simulink model "drone_sim"  (R2022b)
settings: Solver=VariableStepAuto  StartTime=0.0  StopTime=10  RelTol=1e-3
values from neighbouring files (symbols this model uses):
  attitude_0 = [pi/2;pi/2;pi/2;1]    [drone.m]
  g = 9.81    [drone.m]
  k = 1    [drone.m]
  p0 = [0;0;0]    [drone.m]    (also in drone_2.m)
  tau_a = 0.05    [drone.m]
  tau_phi = 0.18    [drone.m]
  tau_psi = 0.56    [drone.m]
  tau_theta = 0.18    [drone.m]
  v0 = [0;0;0]    [drone.m]    (also in drone_2.m)
libraries: slpidlib x4
settings Model: Creator=simonecarena  LastModifiedBy=simonecarena

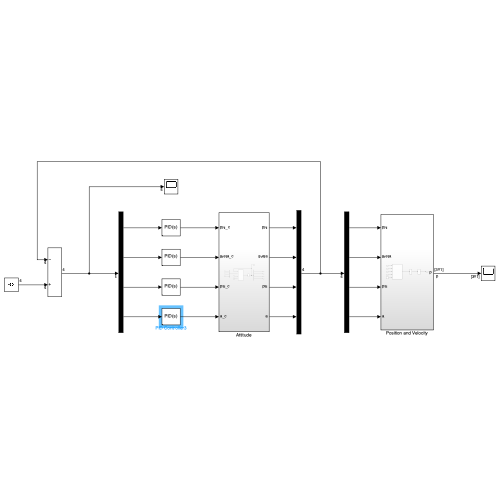
[thumbnail: Simulink's stored preview of the top-level diagram]
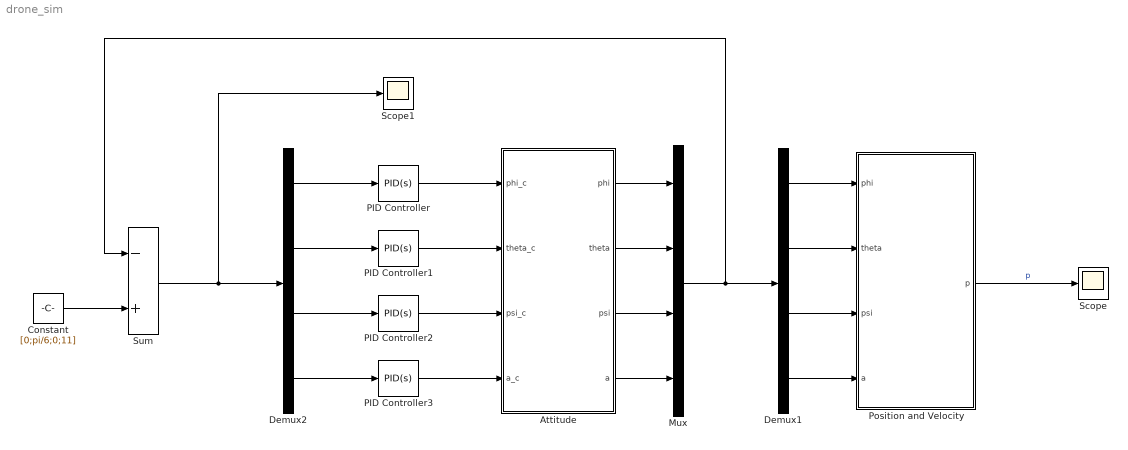
== system drone_sim ==
  Attitude : Subsystem
  Constant : Constant  Value=[0;pi/6;0;11]
  Demux1 : Demux
  Demux2 : Demux
  Mux : Mux
  PID Controller{,1..3} (4 alike) : slpidlib/PID Controller  Controller=PID  Form=Parallel  TimeDomain=Continuous-time  UseExternalTs=off  SampleTime=-1  IntegratorMethod=Forward Euler  FilterMethod=Forward Euler  ControllerParametersSource=internal  P=1  I=0  UseKiTs=off  D=1  N=100  UseFilter=on  TunerSelectOption=Transfer Function Based (PID Tuner App)  InitialConditionSource=internal  InitialConditionForIntegrator=0  InitialConditionForFilter=0  DifferentiatorICPrevScaledInput=0  ExternalReset=none  TrackingMode=off  Kt=1  LimitOutput=off  SatLimitsSource=internal  UpperSaturationLimit=inf  LowerSaturationLimit=-inf  LinearizeAsGain=on  AntiWindupMode=none  Kb=1  LimitIntegrator=off  UpperIntegratorSaturationLimit=inf  LowerIntegratorSaturationLimit=-inf  POutMin=[]  POutMax=[]  IOutMin=[]  IOutMax=[]  DOutMin=[]  DOutMax=[]  NOutMin=[]  NOutMax=[]  SumOutMin=[]  SumOutMax=[]  SaturationOutMin=[]  SaturationOutMax=[]  PParamMin=[]  PParamMax=[]  IParamMin=[]  IParamMax=[]  DParamMin=[]  DParamMax=[]  NParamMin=[]  NParamMax=[]  KbParamMin=[]  KbParamMax=[]  KtParamMin=[]  KtParamMax=[]  KbOutMin=[]  KbOutMax=[]  KtOutMin=[]  KtOutMax=[]  IntegratorOutMin=[]  IntegratorOutMax=[]  FilterOutMin=[]  FilterOutMax=[]  SumI1OutMin=[]  SumI1OutMax=[]  SumI2OutMin=[]  SumI2OutMax=[]  SumI3OutMin=[]  SumI3OutMax=[]  SumI4OutMin=[]  SumI4OutMax=[]  SumDOutMin=[]  SumDOutMax=[]  DifferentiatorOutMin=[]  DifferentiatorOutMax=[]  FilterDiffOutCoefMin=[]  FilterDiffOutCoefMax=[]  ReciprocalOutMin=[]  ReciprocalOutMax=[]  SumDenOutMin=[]  SumDenOutMax=[]  SumNumOutMin=[]  SumNumOutMax=[]  DivideOutMin=[]  DivideOutMax=[]  UdiffTsProdOutMin=[]  UdiffTsProdOutMax=[]  NTsProdOutMin=[]  NTsProdOutMax=[]  UintegralTsProdOutMin=[]  UintegralTsProdOutMax=[]  UngainTsProdOutMin=[]  UngainTsProdOutMax=[]  ClampingZeroOutDataTypeStr=Inherit: Inherit via back propagation  ClampingZeroOutMin=[]  ClampingZeroOutMax=[]  FilterDenConstantOutDataTypeStr=Inherit: Inherit via back propagation  FilterDenConstantOutMin=[]  FilterDenConstantOutMax=[]  PCopyOutDataTypeStr=Inherit: Inherit via back propagation  PCopyOutMin=[]  PCopyOutMax=[]  NCopyOutDataTypeStr=Inherit: Inherit via back propagation  NCopyOutMin=[]  NCopyOutMax=[]  IntegratorContinuousStateAttributes=''  IntegratorStateMustResolveToSignalObject=off  IntegratorRTWStateStorageClass=Auto  FilterContinuousStateAttributes=''  FilterStateMustResolveToSignalObject=off  FilterRTWStateStorageClass=Auto  ParallelPVariant=InternalParameters  IdealPVariant=Disabled  IVariant=InternalParameters  DVariant=InternalParameters  IntegratorVariant=Continuous  SatVariant=Disabled  AWVariant=Passthrough  PCopyVariant=Disabled  TRVariant=Disabled  FdbkBlocksVariant=Forward  IdealPFdbkVariant=Disabled  SatFdbkVariant=Disabled  DerivativeFilterVariant=ContFilter  NVariant=InternalParameters  NCopyVariant=Disabled  FilterICVariant=InternalICsFilter  IntegratorICVariant=InternalICs  ExternalResetVariant=Disabled  TRSumVariant=Passthrough  SumFdbkVariant=Disabled  SumVariant=Sum_PID  TsampFilterVariant=InternalTs  TsampNgainVariant=Passthrough  TsampIntegralVariant=Passthrough  ExternalSaturationOutDataTypeStr=Inherit: Same as second input
  Position and Velocity : Subsystem
  Scope : Scope
  Scope1 : Scope
  Sum : Sum  Inputs=-+
  wires:
  Position and Velocity/1(p) -> Scope/1  "p"
  PID Controller/1 -> Attitude/1(phi_c)
  PID Controller1/1 -> Attitude/2(theta_c)
  PID Controller2/1 -> Attitude/3(psi_c)
  PID Controller3/1 -> Attitude/4(a_c)
  Mux/1 -> Sum/1, Demux1/1
  Attitude/1(phi) -> Mux/1
  Attitude/2(theta) -> Mux/2
  Attitude/3(psi) -> Mux/3
  Attitude/4(a) -> Mux/4
  Demux1/1 -> Position and Velocity/1(phi)
  Demux1/2 -> Position and Velocity/2(theta)
  Demux1/3 -> Position and Velocity/3(psi)
  Demux1/4 -> Position and Velocity/4(a)
  Constant/1 -> Sum/2
  Sum/1 -> Scope1/1, Demux2/1
  Demux2/1 -> PID Controller/1
  Demux2/2 -> PID Controller1/1
  Demux2/3 -> PID Controller2/1
  Demux2/4 -> PID Controller3/1

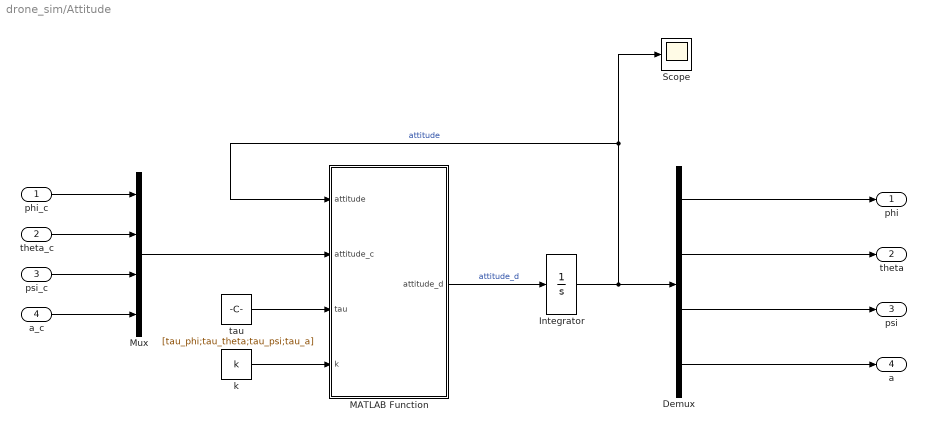
== system drone_sim/Attitude ==
  phi_c : Inport
  theta_c : Inport  Port=2
  psi_c : Inport  Port=3
  a_c : Inport  Port=4
  Demux : Demux
  Integrator : Integrator  InitialCondition=attitude_0
  MATLAB Function : MATLAB Function  TreatAsAtomicUnit=on
  Mux : Mux
  Scope : Scope
  k : Constant  Value=k
  tau : Constant  Value=[tau_phi;tau_theta;tau_psi;tau_a]
  phi : Outport
  theta : Outport  Port=2
  psi : Outport  Port=3
  a : Outport  Port=4
  wires:
  MATLAB Function/1(attitude_d) -> Integrator/1  "attitude_d"
  Integrator/1 -> Scope/1, MATLAB Function/1(attitude), Demux/1  "attitude"
  Demux/1 -> phi/1
  Demux/2 -> theta/1
  Demux/3 -> psi/1
  Demux/4 -> a/1
  phi_c/1 -> Mux/1
  theta_c/1 -> Mux/2
  psi_c/1 -> Mux/3
  a_c/1 -> Mux/4
  Mux/1 -> MATLAB Function/2(attitude_c)
  tau/1 -> MATLAB Function/3(tau)
  k/1 -> MATLAB Function/4(k)

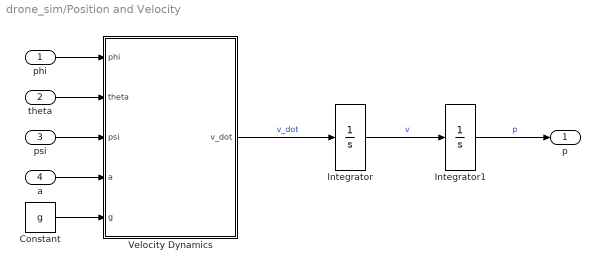
== system drone_sim/Position and Velocity ==
  phi : Inport
  theta : Inport  Port=2
  psi : Inport  Port=3
  a : Inport  Port=4
  Constant : Constant  Value=g
  Integrator : Integrator  InitialCondition=v0
  Integrator1 : Integrator  InitialCondition=p0
  Velocity Dynamics : MATLAB Function  TreatAsAtomicUnit=on
  p : Outport
  wires:
  theta/1 -> Velocity Dynamics/2(theta)
  psi/1 -> Velocity Dynamics/3(psi)
  phi/1 -> Velocity Dynamics/1(phi)
  a/1 -> Velocity Dynamics/4(a)
  Velocity Dynamics/1(v_dot) -> Integrator/1  "v_dot"
  Constant/1 -> Velocity Dynamics/5(g)
  Integrator/1 -> Integrator1/1  "v"
  Integrator1/1 -> p/1  "p"

== matlab function drone_sim/Attitude/MATLAB Function ==
  data: attitude input; attitude_d output; attitude_c input; tau input; k input
function attitude_d = fcn(attitude, attitude_c, tau, k)

    attitude_d = zeros(4,1);

    attitude_d = diag(-1./tau)*attitude+k/tau*attitude_c;

== matlab function drone_sim/Position and Velocity/Velocity Dynamics ==
  data: phi input; v_dot output; theta input; psi input; a input; g input
function v_dot = fcn(phi, theta, psi, a, g)

    v_dot = [
        sin(phi)*sin(psi)+cos(phi)*sin(theta)*cos(psi);
        -sin(phi)*cos(psi)+cos(phi)*sin(theta)*sin(psi);
        cos(phi)*cos(theta)
    ]*a - g*[0;0;1];
